simulink model "Angulo"  (R2022a)
settings: Solver=FixedStepAuto  StartTime=0.0  StopTime=inf  RelTol=1e-3
model workspace (MAT data in the model file):
  Param = Simulink.Parameter
  Param.Value = 90
  Param.DataType = 'auto'
  Param.Complexity = 'real'
  Param.Dimensions = [1 1]
  SL_ROS_VariableLengthArrays_MaxSizes.CommonInfo.ArrayTruncateAction = 'EmitWarning'
  SL_ROS_VariableLengthArrays_MaxSizes.MsgTypeMap = containers.Map
  SL_ROS_VariableLengthArrays_MaxSizes.MsgTypeMap.serialization.keys = {'sensor_msgs/LaserScan'}
  SL_ROS_VariableLengthArrays_MaxSizes.MsgTypeMap.serialization.values{1}(1).PropertyName = 'intensities'
  SL_ROS_VariableLengthArrays_MaxSizes.MsgTypeMap.serialization.values{1}(1).DataType = 'single'
  SL_ROS_VariableLengthArrays_MaxSizes.MsgTypeMap.serialization.values{1}(1).MaxLength = 360
  SL_ROS_VariableLengthArrays_MaxSizes.MsgTypeMap.serialization.values{1}(2).PropertyName = 'ranges'
  SL_ROS_VariableLengthArrays_MaxSizes.MsgTypeMap.serialization.values{1}(2).DataType = 'single'
  SL_ROS_VariableLengthArrays_MaxSizes.MsgTypeMap.serialization.values{1}(2).MaxLength = 360
  SL_ROS_VariableLengthArrays_MaxSizes.MsgTypeMap.serialization.uniformity = 0
  SL_ROS_VariableLengthArrays_MaxSizes.MsgTypeMap.serialization.keyType = 'char'
  SL_ROS_VariableLengthArrays_MaxSizes.MsgTypeMap.serialization.valueType = 'any'
undefined symbols (not defined in the file): angular, header, linear, temperature
libraries: ros2lib x7, dspstat3 x2, simulink_extras x1
settings Model: Creator=Francisco  LastModifiedBy=Francisco
settings OptimizationCC: EnhancedBackFolding=on  PassReuseOutputArgsAs=Individual arguments  ZeroExternalMemoryAtStartup=off  ZeroInternalMemoryAtStartup=off  MaxStackSize=64  OptimizeBlockOrder=speed  DifferentSizesBufferReuse=on  OptimizationCustomize=off  EfficientTunableParamExpr=on
settings DebuggingCC: ParameterTunabilityLossMsg=error
settings SFSimCC: MATLABDynamicMemAlloc=off
settings RTWCC: SystemTargetFile=ert.tlc  HardwareBoard=Robot Operating System 2 (ROS 2)  TLCOptions="-aInlineSetEventsForThisBaseRateFcn=TLC_FALSE -aSuppressMultiTaskScheduler=TLC_FALSE  -aRateBasedStepFcn=0"  TemplateMakefile=ert_default_tmf  Toolchain=Colcon Tools  TargetLang=C++
settings CodeAppCC: ForceParamTrailComments=on  IgnoreCustomStorageClasses=off  OperatorAnnotations=on  SimulinkDataObjDesc=on  SFDataObjDesc=on  InsertBlockDesc=on
settings ERTTargetCC: CodeInterfacePackaging=C++ class  SupportContinuousTime=on  RootIOFormat=Structure reference

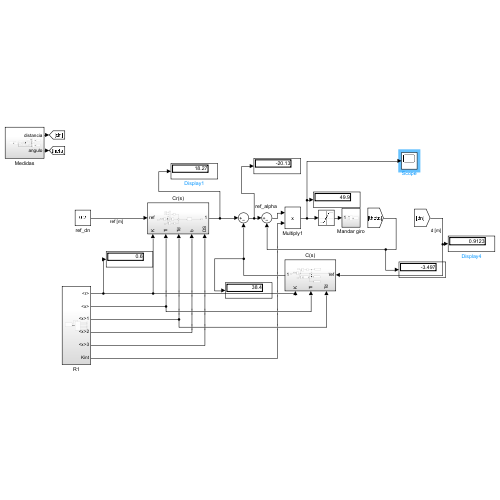
[thumbnail: Simulink's stored preview of the top-level diagram]
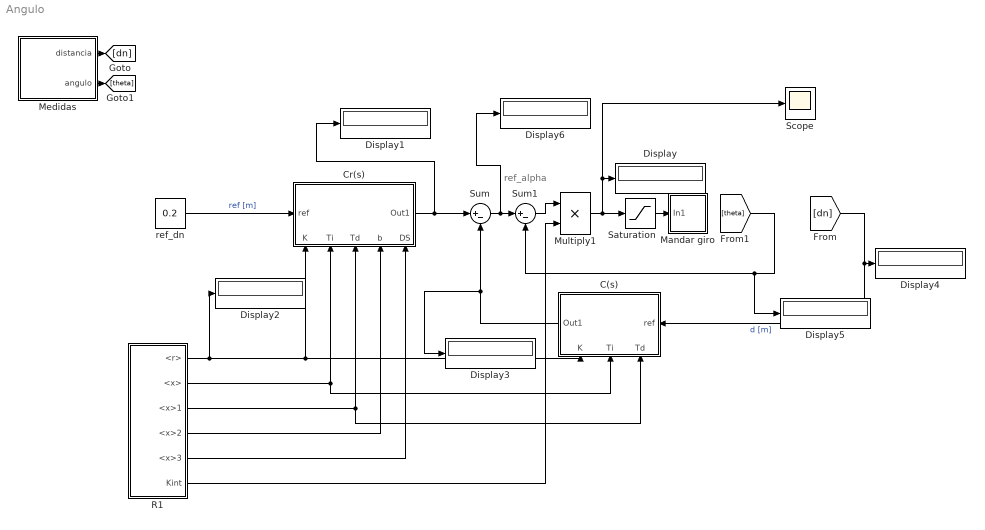
== system Angulo ==
  note: ref_alpha
  C(s) : Subsystem
      settings: PortSchema="{\"entries\":[{\"content\":{\"sides\":[{\"content\":{\"connectorIds\":[\"In1\"]},\"type\":\"ConnectorPlacement.EquallySpacedRectSide\",\"uuid\":\"394aa06e-278b-4cf5-817b-3cfa1141fba0\"},{\"content\":{\"connectorIds\":[\"Out1\"],\"side\":\"RIGHT\"},\"type\":\"ConnectorPlacement.EquallySpacedRectSide\",\"uuid\":\"0e5f8416-e921-47f8-867e-c9c380a043c0\"},{\"content\":{\"connectorIds\":[\"In2\",\"In3\",\"In4\"],\"side\":\"TOP\"},\"type\":\"ConnectorPlacement.EquallySpacedRectSide\",\"uuid\":\"8a994927-802b-4b1c-973c-ad4840c3f2b4\"},{\"content\":{\"connectorIds\":[],\"side\":\"BOTTOM\"},\"type\":\"ConnectorPlacement.EquallySpacedRectSide\",\"uuid\":\"54c24353-aa9e-4228-8783-90e7d41035bc\"}]},\"type\":\"ConnectorPlacement.EquallySpacedConnector\",\"uuid\":\"debdf9f7-4d5e-43e8-b321-9f3f69ff3cfc\"}],\"packageUris\":[\"http://schema.mathworks.com/mf0/Connector/R2020b\"],\"version\":\"1.0\"}"
  Cr(s) : Subsystem
      settings: PortSchema="{\"entries\":[{\"content\":{\"sides\":[{\"content\":{\"connectorIds\":[\"In1\"]},\"type\":\"ConnectorPlacement.EquallySpacedRectSide\",\"uuid\":\"394aa06e-278b-4cf5-817b-3cfa1141fba0\"},{\"content\":{\"connectorIds\":[\"Out1\"],\"side\":\"RIGHT\"},\"type\":\"ConnectorPlacement.EquallySpacedRectSide\",\"uuid\":\"0e5f8416-e921-47f8-867e-c9c380a043c0\"},{\"content\":{\"connectorIds\":[],\"side\":\"TOP\"},\"type\":\"ConnectorPlacement.EquallySpacedRectSide\",\"uuid\":\"8a994927-802b-4b1c-973c-ad4840c3f2b4\"},{\"content\":{\"connectorIds\":[\"In2\",\"In3\",\"In4\",\"In5\",\"In6\"],\"side\":\"BOTTOM\"},\"type\":\"ConnectorPlacement.EquallySpacedRectSide\",\"uuid\":\"54c24353-aa9e-4228-8783-90e7d41035bc\"}]},\"type\":\"ConnectorPlacement.EquallySpacedConnector\",\"uuid\":\"debdf9f7-4d5e-43e8-b321-9f3f69ff3cfc\"}],\"packageUris\":[\"http://schema.mathworks.com/mf0/Connector/R2020b\"],\"version\":\"1.0\"}"
  Display{,1..6} (7 alike) : Display
  Mandar giro : Subsystem
  Medidas : Subsystem
  Multiply1 : Product
  R1 : Subsystem
  Saturation : Saturate  UpperLimit=100  LowerLimit=-100  LinearizeAsGain=off
  Scope : Scope
  Sum : Sum  Inputs=|+-
  Sum1 : Sum  Inputs=|+-
  ref_dn : Constant  Value=0.2
  wires:
  Cr(s)/1(Out1) -> Display1/1, Sum/1
  Sum/1 -> Display6/1, Sum1/1
  [dn] -> Display4/1, C(s)/1(ref)  "d [m]"
  Saturation/1 -> Mandar giro/1(In1)
  Medidas/1(distancia) -> [dn]
  Medidas/2(angulo) -> [theta]
  Sum1/1 -> Multiply1/1
  Multiply1/1 -> Scope/1, Display/1, Saturation/1
  [theta] -> Display5/1, Sum1/2
  C(s)/1(Out1) -> Sum/2, Display3/1
  R1/4(<x>2) -> Cr(s)/5(b)
  R1/5(<x>3) -> Cr(s)/6(DS)
  R1/3(<x>1) -> C(s)/2(Td), Cr(s)/4(Td)
  R1/2(<x>) -> C(s)/3(Ti), Cr(s)/3(Ti)
  ref_dn/1 -> Cr(s)/1(ref)  "ref [m]"
  R1/6(Kint) -> Multiply1/2
  R1/1(<r>) -> Display2/1, C(s)/4(K), Cr(s)/2(K)

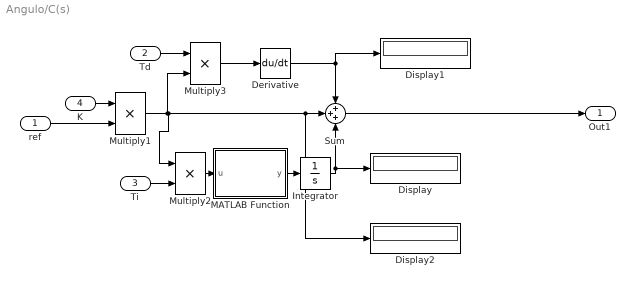
== system Angulo/C(s) ==
  ref : Inport
  Td : Inport  Port=2
  Ti : Inport  Port=3
  K : Inport  Port=4
  Derivative : Derivative
  Display : Display
  Display1 : Display
  Display2 : Display
  Integrator : Integrator  LimitOutput=on  UpperSaturationLimit=100  LowerSaturationLimit=-100
  MATLAB Function : MATLAB Function  TreatAsAtomicUnit=on
  Multiply1 : Product
  Multiply2 : Product
  Multiply3 : Product
  Sum : Sum  Inputs=+++
  Out1 : Outport
  wires:
  Multiply2/1 -> MATLAB Function/1(u)
  Td/1 -> Multiply3/1
  Ti/1 -> Multiply2/2
  Multiply1/1 -> Display2/1, Sum/2, Multiply2/1, Multiply3/2
  Multiply3/1 -> Derivative/1
  Derivative/1 -> Sum/1, Display1/1
  K/1 -> Multiply1/1
  Integrator/1 -> Display/1, Sum/3
  ref/1 -> Multiply1/2
  Sum/1 -> Out1/1
  MATLAB Function/1(y) -> Integrator/1

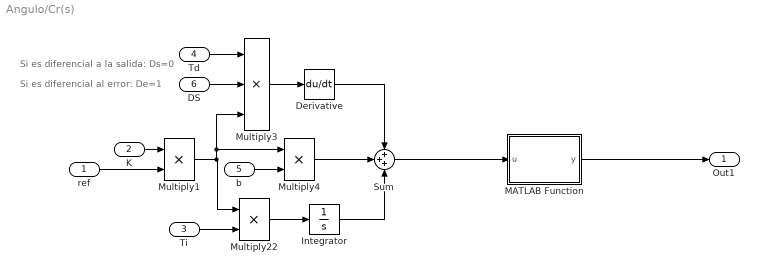
== system Angulo/Cr(s) ==
  note: Si es diferencial a la salida: Ds=0
  note: Si es diferencial al error: De=1
  ref : Inport
  K : Inport  Port=2
  Ti : Inport  Port=3
  Td : Inport  Port=4
  b : Inport  Port=5
  DS : Inport  Port=6
  Derivative : Derivative
  Integrator : Integrator  LimitOutput=on  UpperSaturationLimit=100  LowerSaturationLimit=-100
  MATLAB Function : MATLAB Function  TreatAsAtomicUnit=on
  Multiply1 : Product
  Multiply22 : Product
  Multiply3 : Product  Inputs=3
  Multiply4 : Product
  Sum : Sum  Inputs=+++
  Out1 : Outport
  wires:
  Multiply22/1 -> Integrator/1
  Td/1 -> Multiply3/1
  Ti/1 -> Multiply22/2
  Multiply1/1 -> Multiply3/3, Multiply4/1, Multiply22/1
  Multiply3/1 -> Derivative/1
  Derivative/1 -> Sum/1
  K/1 -> Multiply1/1
  Integrator/1 -> Sum/3
  ref/1 -> Multiply1/2
  Sum/1 -> MATLAB Function/1(u)
  Multiply4/1 -> Sum/2
  b/1 -> Multiply4/2
  DS/1 -> Multiply3/2
  MATLAB Function/1(y) -> Out1/1

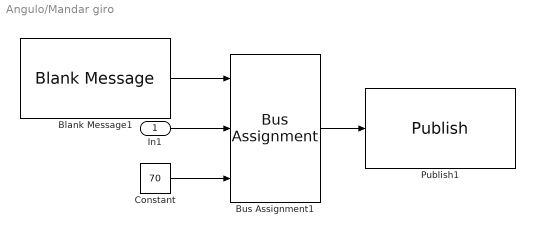
== system Angulo/Mandar giro ==
  In1 : Inport
  Blank Message1 : ros2lib/Blank Message  messageClass=Message  entityType=geometry_msgs/Twist  messageType=geometry_msgs/Twist  SampleTime=inf
      settings: SourceProductBaseCode=RR
  Bus Assignment1 : BusAssignment  AssignedSignals=angular.z,linear.x
  Constant : Constant  Value=70
  Publish1 : ros2lib/Publish  topicSource=Select from ROS network  topic=/cmd_vel  messageType=geometry_msgs/Twist  QOSHistory=Keep last  QOSDepth=1  QOSReliability=Reliable  QOSDurability=Volatile
      settings: SourceProductBaseCode=RR
  wires:
  Bus Assignment1/1 -> Publish1/1
  Blank Message1/1 -> Bus Assignment1/1
  In1/1 -> Bus Assignment1/2
  Constant/1 -> Bus Assignment1/3

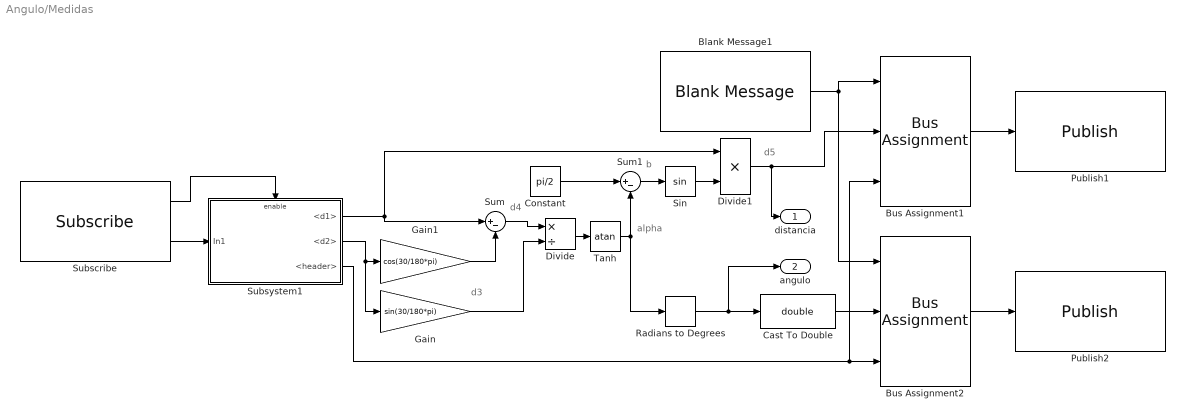
== system Angulo/Medidas ==
  note: d5
  note: b
  note: alpha
  note: d3
  note: d4
  Blank Message1 : ros2lib/Blank Message  messageClass=Message  entityType=sensor_msgs/Temperature  messageType=sensor_msgs/Temperature  SampleTime=1/360
      settings: SourceProductBaseCode=RR
  Bus Assignment1 : BusAssignment  AssignedSignals=temperature,header
  Bus Assignment2 : BusAssignment  AssignedSignals=temperature,header
  Cast To Double : DataTypeConversion  OutDataTypeStr=double  SaturateOnIntegerOverflow=off  RndMeth=Floor
  Constant : Constant  Value=pi/2
  Divide : Product  Inputs=*/
  Divide1 : Product  Inputs=**
  Gain : Gain  Gain=sin(30/180*pi)
  Gain1 : Gain  Gain=cos(30/180*pi)
  Publish1 : ros2lib/Publish  topicSource=Specify your own  topic=/distanciaPared  messageType=sensor_msgs/Temperature  QOSHistory=Keep last  QOSDepth=1  QOSReliability=Reliable  QOSDurability=Volatile
      settings: SourceProductBaseCode=RR
  Publish2 : ros2lib/Publish  topicSource=Specify your own  topic=/anguloPared  messageType=sensor_msgs/Temperature  QOSHistory=Keep last  QOSDepth=1  QOSReliability=Reliable  QOSDurability=Volatile
      settings: SourceProductBaseCode=RR
  Radians to Degrees : simulink_extras/Transformations/Radians to Degrees
  Sin : Trigonometry
  Subscribe : ros2lib/Subscribe  topicSource=Select from ROS network  topic=/scan  messageType=sensor_msgs/LaserScan  sampleTime=-1  QOSHistory=Keep last  QOSDepth=10  QOSReliability=Best effort  QOSDurability=Volatile
      settings: SourceProductBaseCode=RR
  Subsystem1 : Subsystem
  Sum : Sum  Inputs=|+-
  Sum1 : Sum  Inputs=|+-
  Tanh : Trigonometry  Operator=atan
  distancia : Outport
  angulo : Outport  Port=2
  wires:
  Subscribe/1 -> Subsystem1/Enable
  Constant/1 -> Sum1/1
  Subsystem1/1(<d1>) -> Sum/1, Divide1/1
  Subsystem1/2(<d2>) -> Gain/1, Gain1/1
  Subscribe/2 -> Subsystem1/1(In1)
  Cast To Double/1 -> Bus Assignment2/2
  Gain/1 -> Divide/2
  Sum/1 -> Divide/1
  Gain1/1 -> Sum/2
  Sin/1 -> Divide1/2
  Tanh/1 -> Sum1/2, Radians to Degrees/1
  Divide/1 -> Tanh/1
  Radians to Degrees/1 -> angulo/1, Cast To Double/1
  Subsystem1/3(<header>) -> Bus Assignment1/3, Bus Assignment2/3
  Sum1/1 -> Sin/1
  Bus Assignment1/1 -> Publish1/1
  Bus Assignment2/1 -> Publish2/1
  Blank Message1/1 -> Bus Assignment2/1, Bus Assignment1/1
  Divide1/1 -> distancia/1, Bus Assignment1/2

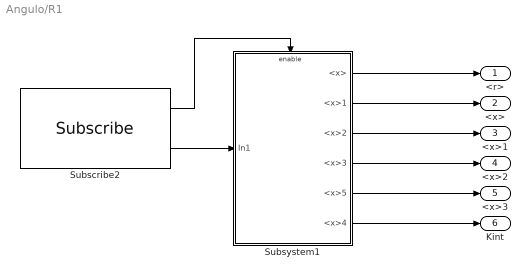
== system Angulo/R1 ==
  Subscribe2 : ros2lib/Subscribe  topicSource=Specify your own  topic=/control  messageType=geometry_msgs/Twist  sampleTime=-1  QOSHistory=Keep last  QOSDepth=1  QOSReliability=Reliable  QOSDurability=Volatile
      settings: SourceProductBaseCode=RR
  Subsystem1 : Subsystem
  <r> : Outport
  <x> : Outport  Port=2
  <x>1 : Outport  Port=3
  <x>2 : Outport  Port=4
  <x>3 : Outport  Port=5
  Kint : Outport  Port=6
  wires:
  Subscribe2/1 -> Subsystem1/Enable
  Subscribe2/2 -> Subsystem1/1(In1)
  Subsystem1/1(<x>) -> <r>/1
  Subsystem1/4(<x>3) -> <x>2/1
  Subsystem1/2(<x>1) -> <x>/1
  Subsystem1/5(<x>5) -> <x>3/1
  Subsystem1/3(<x>2) -> <x>1/1
  Subsystem1/6(<x>4) -> Kint/1

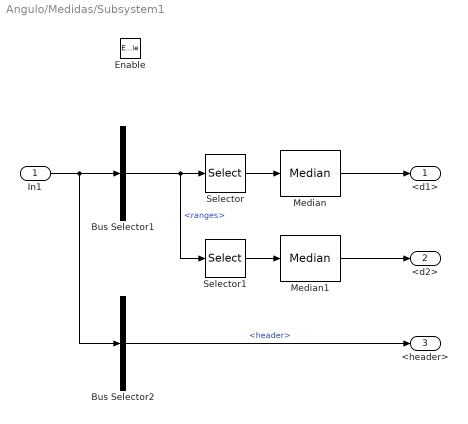
== system Angulo/Medidas/Subsystem1 ==
  In1 : Inport
  Enable : EnablePort
  Bus Selector1 : BusSelector  OutputSignals=ranges
  Bus Selector2 : BusSelector  OutputSignals=header
  Median : dspstat3/Median  sortAlg=Quick sort  directionMode=Each column  dimension=1  roundingMode=Floor  overflowMode=off  accumDataTypeStr=Inherit: Same as product output  accumLastDataTypeStr=Inherit: Same as product output  outputDataTypeStr=Inherit: Same as accumulator  outputMin=[]  outputMax=[]  outputLastDataTypeStr=Inherit: Same as accumulator
      settings: SourceProductBaseCode=DS  allowOverrides=off
  Median1 : dspstat3/Median  sortAlg=Quick sort  directionMode=Each column  dimension=1  roundingMode=Floor  overflowMode=off  accumDataTypeStr=Inherit: Same as product output  accumLastDataTypeStr=Inherit: Same as product output  outputDataTypeStr=Inherit: Same as accumulator  outputMin=[]  outputMax=[]  outputLastDataTypeStr=Inherit: Same as accumulator
      settings: SourceProductBaseCode=DS  allowOverrides=off
  Selector : Selector  IndexMode=Zero-based  InputPortWidth=360  IndexOptions=Index vector (dialog)  Indices=[88:92]  OutputSizes=1
  Selector1 : Selector  IndexMode=Zero-based  InputPortWidth=360  IndexOptions=Index vector (dialog)  Indices=[118:122]  OutputSizes=1
  <d1> : Outport
  <d2> : Outport  Port=2
  <header> : Outport  Port=3
  wires:
  In1/1 -> Bus Selector2/1, Bus Selector1/1
  Bus Selector1/1 -> Selector1/1, Selector/1  "<ranges>"
  Selector/1 -> Median/1
  Selector1/1 -> Median1/1
  Median/1 -> <d1>/1
  Median1/1 -> <d2>/1
  Bus Selector2/1 -> <header>/1  "<header>"

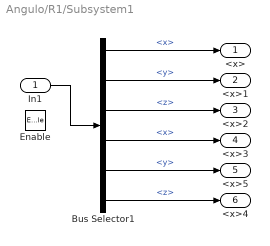
== system Angulo/R1/Subsystem1 ==
  In1 : Inport
  Enable : EnablePort
  Bus Selector1 : BusSelector  OutputSignals=linear.x,linear.y,linear.z,angular.x,angular.y,angular.z
  <x> : Outport
  <x>1 : Outport  Port=2
  <x>2 : Outport  Port=3
  <x>3 : Outport  Port=4
  <x>5 : Outport  Port=5
  <x>4 : Outport  Port=6
  wires:
  In1/1 -> Bus Selector1/1
  Bus Selector1/1 -> <x>/1  "<x>"
  Bus Selector1/2 -> <x>1/1  "<y>"
  Bus Selector1/3 -> <x>2/1  "<z>"
  Bus Selector1/4 -> <x>3/1  "<x>"
  Bus Selector1/5 -> <x>5/1  "<y>"
  Bus Selector1/6 -> <x>4/1  "<z>"

== matlab function Angulo/Cr(s)/MATLAB Function ==
  data: u input; y output
function y = fcn(u)
% Verify that the input is not a number. If it is true, the function output will be made equal to 0 or eps. This can be necessary when a signal passes through a function that uses an integral/derivative.
if isnan(u) || isinf(u)
u=0; % Or eps (to avoid division by zero)
end
y = u;

== matlab function Angulo/C(s)/MATLAB Function ==
  data: u input; y output
function y = fcn(u)
% Verify that the input is not a number. If it is true, the function output will be made equal to 0 or eps. This can be necessary when a signal passes through a function that uses an integral/derivative.
if isnan(u) || isinf(u)
u=0; % Or eps (to avoid division by zero)
end
y = u;
